simulink model "Main_v2"  (R2022b)
settings: Solver=ode23  StartTime=0.0  StopTime=sim_time-0.02
values from neighbouring files (symbols this model uses):
  bike_model = 1    [Main_sim.m]    (also in Startup_Script.m; Startup_Script_v2.m)
  bike_params = LoadBikeParameters(bike)    [Kalman_offline.m]    (also in Main_sim.m; Startup_Script.m; Startup_Script_v2.m; Startup_labview.m)
  C1 = [1 0 0 0 0 0 0 ... (first row only)    [Kalman_offline.m]    (also in Main_sim.m; Startup_Script.m; Startup_Script_v2.m; Startup_labview.m)
  counter = (Ts_GPS / Ts) - 1    (= 9)    [Kalman_offline.m]    (also in Main_sim.m; Startup_Script.m; Startup_Script_v2.m; Startup_labview.m)
  D_balancing_inner = 0    [Main_sim.m]    (also in Startup_Script.m; Startup_Script_v2.m; Startup_labview.m)
  D_balancing_outer = 0.0    (= 0)    [Main_sim.m]    (also in Startup_Script.m; Startup_Script_v2.m; Startup_labview.m)
  e1_max = abs(-k2*e2_max/k1)    [Main_sim.m]    (also in Startup_Script.m; Startup_Script_v2.m; Startup_labview.m)
  g = -9.81    [Kalman_offline.m]    (also in Main_sim.m = 9.81; Startup_Script.m = 9.81; Startup_Script_v2.m = 9.81; Startup_labview.m = 9.81)
  hor_dis = 10    [Main_sim.m]    (also in Startup_Script.m = 1; Startup_Script_v2.m = 1)
  I_balancing_inner = 0    [Main_sim.m]    (also in Startup_Script.m; Startup_Script_v2.m; Startup_labview.m)
  I_balancing_outer = 0.0    (= 0)    [Main_sim.m]    (also in Startup_Script.m; Startup_Script_v2.m; Startup_labview.m)
  initial_state_estimate = initial_state    [Main_sim.m]    (also in Startup_Script.m; Startup_Script_v2.m)
  k1 = K(1)    [Main_sim.m]    (also in Startup_Script.m; Startup_Script_v2.m; Startup_labview.m)
  k2 = K(2)    [Main_sim.m]    (also in Startup_Script.m; Startup_Script_v2.m; Startup_labview.m)
  Kalman_gain1 = Kalman_gain1'    [Kalman_offline.m]    (also in Main_sim.m; Startup_Script.m; Startup_Script_v2.m; Startup_labview.m)
  Kalman_gain2 = Kalman_gain2'    [Kalman_offline.m]    (also in Main_sim.m = Kalman_gain1(4:7,3:7); Startup_Script.m; Startup_Script_v2.m; Startup_labview.m = Kalman_gain1(4:7,3:7))
  linearized_sys = ss(A,B,C,D)    [Startup_Script_v2.m]
  P_balancing_inner = 3    [Main_sim.m]    (also in Startup_Script.m; Startup_Script_v2.m; Startup_labview.m = 1)
  P_balancing_outer = 1.3    [Main_sim.m]    (also in Startup_Script.m; Startup_Script_v2.m; Startup_labview.m = 1.75)
  Psiref = psiref'    [ReferenceGenerator.m]
  ref_dis = 0.01    [Main_sim.m]    (also in Startup_Script.m; Startup_Script_v2.m)
  ref_start_idx = 2    [Main_sim.m]    (also in Startup_Script.m; Startup_Script_v2.m)
  Ts = 0.01    [Kalman_offline.m]    (also in Main_sim.m; Startup_Script.m; Startup_Script_v2.m; Startup_labview.m)
  v = 3    [Main_sim.m]    (also in Startup_Script.m; Startup_Script_v2.m; Startup_labview.m = 2; Test_ss.m)
  Xref = xref'    [ReferenceGenerator.m]
  Yref = yref'    [ReferenceGenerator.m]
undefined symbols (not defined in the file or in its folder): initial_state, pert_deltadot_state, pert_deltadot_state_fun, pert_phidot_state, pert_phidot_state_fun
libraries: eeGeneralControl x3, slpidlib x2, simulink x2, cstblocks x1
(part 2 of 2)

== matlab function Main_v2/State estimator/Linearized Bicycle Model on Constant Velocity ==
  data: Est_States input; dot_delta_e input; y input; Kalman_gain1 input; Kalman_gain2 input; bike_params input; Ts input; Est_states output; v input; flag input
function Est_states  = fcn(Est_States, dot_delta_e, y, Kalman_gain1, Kalman_gain2, bike_params,Ts,v,flag)
% description 
% Inputs
%   Est_States := [X Y psi phi phi_dot delta_e v] are global at time t 
%   dot_delta_e := effective steering rate
%   y := measurement vector
%   Kalman_gain1 := Computed state_feedback gain including GPS meas
%   Kalman_gain2 := Computed state_feedback gain excluding GPS meas
%   bike_params := vector of bike parameters + gravity
%   Ts := Estimator sampling rate
%   v := constant velocity
%   flag := [0-1] increasing counter reseted at 1. When flag == 0 means
%           that GPS measurement is available
%
% Outputs
%   Est_states : = [X Y psi phi phi_dot delta_e v] global at time t+1

% Unpacked bike_params
    g = bike_params(1);
    h = bike_params(2);
    b = bike_params(3);
    a = bike_params(4);
    lambda = bike_params(5);
    c = bike_params(6);
    m = bike_params(7);
    h_imu = bike_params(8);

% Paper symbology
    lr = a; % distance from rear wheel center to center of mass
    lf = b-a; % distance from front wheel center to center of mass


% Transform the states to local frame 
    Est_States_l = zeros(7,1);
    
    Est_States_l(1) = Est_States(1) * cos(Est_States(3)) + Est_States(2) * sin(Est_States(3));
    Est_States_l(2) = -Est_States(1) * sin(Est_States(3)) + Est_States(2) * cos(Est_States(3));
    Est_States_l(3) = 0;        % direction of bike is aligned with X local frame
    Est_States_l(4) = Est_States(4);
    Est_States_l(5) = Est_States(5);
    Est_States_l(6) = Est_States(6);
    Est_States_l(7) = Est_States(7);

% Transform measurements to local frame
    y_l = zeros(size(y));

    y_l(1) = y(1) * cos(Est_States(3)) + y(2) * sin(Est_States(3));
    y_l(2) = -y(1) * sin(Est_States(3)) + y(2) * cos(Est_States(3)); 
    y_l(3) = y(3);
    y_l(4) = y(4);
    y_l(5) = y(5);
    y_l(6) = y(6);
    y_l(7) = y(7);


% % Continuous Time update in local frame TODO: x(t+1) = (I+A delta_T)h_hat(t)
%     states_dot = zeros(7,1);
%     
%     states_dot(1) = Est_States(7);
%     states_dot(2) = v * (Est_States_l(3) + (lr/(lr+lf))*Est_States(6) );
%     states_dot(3) = (v/(lr+lf)) * Est_States(6);
%     states_dot(4) = Est_States(5);
%     states_dot(5) = (g/h)*Est_States(4) + ((v^2*h-lr*g*c)/(h*(lr+lf)))*Est_States(6) + ((lr*v)/(h^2*(lr+lf)))*dot_delta_e;
%     states_dot(6) = dot_delta_e;
%     states_dot(7) = 0;
% 
% % Discrete time update in local 
%     Est_States_l = Est_States_l + states_dot * Ts; 

% % C identity is used to see if the code runs
%     sen = zeros(6,1);
%     sen(1)      = States_l(1);  
%     sen(2)      = States_l(2);
%     %sen(3)      = States_l(3);
%     sen(3)      = States_l(4);
%     sen(4)      = States_l(5);
%     sen(5)      = States_l(6);
%     sen(6)      = States_l(7);

% % Transform measurements into local frame to see if code runs
%     meas_l = zeros(6,1);
%     meas_l(1) = meas(1) * cos(States(3)) + meas(2) * sin(States(3));
%     meas_l(2) = -meas(1) * sin(States(3)) + meas(2) * cos(States(3));
%     meas_l(3) = 0;
%     meas_l(3) = meas(3)-States(3);  
%     meas_l(3) = meas(4);
%     meas_l(4) = meas(5);
%     meas_l(5) = meas(6);
%     meas_l(6) = meas(7);
%     meas_l(7) = meas(7);

% Time update in local frame (from t to t+1)
    % A matrix (linear bicycle model with constant velocity)
    A = [0 0 0 0 0 0 1;
         0 0 v 0 0 v*(lr/(lf+lr)) 0;
         0 0 0 0 0 (v/(lr+lf)) 0;
         0 0 0 0 1 0 0;
         0 0 0 (g/h) 0 ((v^2*h-lr*g*c)/(h^2*(lr+lf))) 0;
         0 0 0 0 0 0 0;
         0 0 0 0 0 0 0];
    
    % B matrix (linear bicycle model with constant velocity)
    B = [0 0 0 0 ((lr*v)/(h*(lr+lf))) 1 0]';
    
    % Discretization
    A_d = (eye(size(A))+Ts*A);
    B_d = Ts*B;

    % Time update
     Est_States_l = A_d*Est_States_l + B_d*dot_delta_e;

% Measurement update in local frame
    Est_states_l = zeros(7,1);

    % Sampling differentiation (Sensors rate 100Hz but GPS 10Hz)

    if flag == 0 % GPS sensors included
    
        % Select Kalman Gain
            K = Kalman_gain1;
    
        % C matrix for measurements
            X_GPS       = Est_States_l(1);  
            Y_GPS       = Est_States_l(2);
            a_y         = Est_States_l(6)*((-h_imu*(h*v^2-(g*a*c))*sin(lambda)/(b*h^2))+((v^2*sin(lambda))/(b))) + Est_States_l(4)*(g-((h_imu*g)/(h)))+ (-h_imu*a*v*sin(lambda)/(b*h))*dot_delta_e;
            omega_x     = Est_States_l(5);
            omega_z     = Est_States_l(6)*(v*sin(lambda))/(b);
            delta_enc   = Est_States_l(6);
            v_sens      = Est_States_l(7);
            y_pred = [X_GPS Y_GPS a_y omega_x omega_z delta_enc v_sens]';
    
        % Measurement update
            Est_states_l = Est_States_l + K * (y_l - y_pred);
            
    else % GPS sensors excluded
    
        % Select Kalman Gain
            K = Kalman_gain2;
    
        % C matrix for measurements
            a_y         = Est_States_l(6)*((-h_imu*(h*v^2-(g*a*c))*sin(lambda)/(b*h^2))+((v^2*sin(lambda))/(b))) + Est_States_l(4)*(g-((h_imu*g)/(h)))+ (-h_imu*a*v*sin(lambda)/(b*h))*dot_delta_e;
            omega_x     = Est_States_l(5);
            omega_z     = Est_States_l(6)*(v*sin(lambda))/(b);
            delta_enc   = Est_States_l(6);
            v_sens      = Est_States_l(7);
            y_pred = [a_y omega_x omega_z delta_enc v_sens]';
            
        % Measurement update
        Est_states_l(1) = Est_States_l(1);
        Est_states_l(2) = Est_States_l(2);
        Est_states_l(3) = Est_States_l(3);
        Est_states_l(4) = Est_States_l(4)+ K(1,:) * (y_l(3:7) - y_pred);
        Est_states_l(5) = Est_States_l(5) ;%+ K(2,:) * (y_l(3:7) - y_pred);
        Est_states_l(6) = Est_States_l(6)+ K(3,:) * (y_l(3:7) - y_pred);
        Est_states_l(7) = Est_States_l(7)+ K(4,:) * (y_l(3:7) - y_pred);

%         Est_states_l(4:7) = Est_States_l(4:7) + K * (y_l(3:7) - y_pred);
    end

    % states_l = Kalman_gain * (meas_l - sen);
    % states_l(1) = States_l(1) + Kalman_gain(1,1) * (meas_l(1) - x_m) + Kalman_gain(1,2) * (meas_l(2) - y_m) + Kalman_gain(1,3) * (meas_l(3) - psi_m) + Kalman_gain(1,4) * (meas_l(4) - phi_m) + Kalman_gain(1,5) * (meas_l(5) - dot_phi_m) + Kalman_gain(1,6) * (meas_l(6) - delta_m) + Kalman_gain(1,7) * (meas_l(7) - v_m);
    % states_l(2) = States_l(2) + Kalman_gain(2,1) * (meas_l(1) - x_m) + Kalman_gain(2,2) * (meas_l(2) - y_m) + Kalman_gain(2,3) * (meas_l(3) - psi_m) + Kalman_gain(2,4) * (meas_l(4) - phi_m) + Kalman_gain(2,5) * (meas_l(5) - dot_phi_m) + Kalman_gain(2,6) * (meas_l(6) - delta_m) + Kalman_gain(2,7) * (meas_l(7) - v_m);
    % states_l(3) = States_l(3) + Kalman_gain(3,1) * (meas_l(1) - x_m) + Kalman_gain(3,2) * (meas_l(2) - y_m) + Kalman_gain(3,3) * (meas_l(3) - psi_m) + Kalman_gain(3,4) * (meas_l(4) - phi_m) + Kalman_gain(3,5) * (meas_l(5) - dot_phi_m) + Kalman_gain(3,6) * (meas_l(6) - delta_m) + Kalman_gain(3,7) * (meas_l(7) - v_m);
    % states_l(4) = States_l(4) + Kalman_gain(4,1) * (meas_l(1) - x_m) + Kalman_gain(4,2) * (meas_l(2) - y_m) + Kalman_gain(4,3) * (meas_l(3) - psi_m) + Kalman_gain(4,4) * (meas_l(4) - phi_m) + Kalman_gain(4,5) * (meas_l(5) - dot_phi_m) + Kalman_gain(4,6) * (meas_l(6) - delta_m) + Kalman_gain(4,7) * (meas_l(7) - v_m);
    % states_l(5) = States_l(5) + Kalman_gain(5,1) * (meas_l(1) - x_m) + Kalman_gain(5,2) * (meas_l(2) - y_m) + Kalman_gain(5,3) * (meas_l(3) - psi_m) + Kalman_gain(5,4) * (meas_l(4) - phi_m) + Kalman_gain(5,5) * (meas_l(5) - dot_phi_m) + Kalman_gain(5,6) * (meas_l(6) - delta_m) + Kalman_gain(5,7) * (meas_l(7) - v_m);
    % states_l(6) = States_l(6) + Kalman_gain(6,1) * (meas_l(1) - x_m) + Kalman_gain(6,2) * (meas_l(2) - y_m) + Kalman_gain(6,3) * (meas_l(3) - psi_m) + Kalman_gain(6,4) * (meas_l(4) - phi_m) + Kalman_gain(6,5) * (meas_l(5) - dot_phi_m) + Kalman_gain(6,6) * (meas_l(6) - delta_m) + Kalman_gain(6,7) * (meas_l(7) - v_m);
    % states_l(7) = States_l(7) + Kalman_gain(7,1) * (meas_l(1) - x_m) + Kalman_gain(7,2) * (meas_l(2) - y_m) + Kalman_gain(7,3) * (meas_l(3) - psi_m) + Kalman_gain(7,4) * (meas_l(4) - phi_m) + Kalman_gain(7,5) * (meas_l(5) - dot_phi_m) + Kalman_gain(7,6) * (meas_l(6) - delta_m) + Kalman_gain(7,7) * (meas_l(7) - v_m);

% Transform to global the local states at time t+1 after measurement update
    Est_states = zeros(7,1);
    Est_states(3) = Est_States(3) + Est_states_l(3);    % direction update global
    
    % Change of Coordinates from local to global frame for  states 
    Est_states(1) = Est_states_l(1) * cos(Est_States(3)) - Est_states_l(2) * sin(Est_States(3));
    Est_states(2) = Est_states_l(1) * sin(Est_States(3)) + Est_states_l(2) * cos(Est_States(3));
    Est_states(4) = Est_states_l(4);
    Est_states(5) = Est_states_l(5);
    Est_states(6) = Est_states_l(6);
    Est_states(7) = Est_states_l(7);
    
    % Heading angle between pi and -pi
    Est_states(3) = wrapToPi(Est_states(3));

end

== matlab function Main_v2/Unstable bike model/Track bycicle pose/Derivative of positions ==
  data: Speed input; beta input; psi input; Xdot output; Ydot output
function [Xdot, Ydot]  = fcn(Speed, beta, psi)

Xdot = Speed * cos(psi + beta);
Ydot = Speed * sin(psi + beta);

== matlab function Main_v2/Unstable bike model/Nonlinear Model of the Physical Bicycle/MATLAB Function ==
  data: States input; xdot output; Steering_rate input; Speed input; disturbances input; bike_params input
function xdot = fcn(States, Steering_rate, Speed, disturbances, bike_params)
% Unpacked bike_params
    g = bike_params(1);
    h = bike_params(2);
    b = bike_params(3);
    a = bike_params(4);
    lambda = bike_params(5);
    c = bike_params(6);
    m = bike_params(7);
    h_imu = bike_params(8);

% Paper symbology
    lr = a; % distance from rear wheel center to center of mass
    lf = b-a; % distance from front wheel center to center of mass

d_phidot = disturbances(1);
d_deltadot = disturbances(2);

phi = States(1);
delta = States(2);
phi_d = States(3);

% xdot = [phidot deltadot phiddot]
xdot1 = phi_d + d_phidot;
xdot2 = Steering_rate + d_deltadot;
xdot3 = (g/h)*phi + ((lr*Speed*sin(lambda))/((lr+lf)*h))*Steering_rate + ((h*Speed^2-g*lr*c)/((lr+lf)*h^2))*sin(lambda)*delta;

xdot = [xdot1 xdot2 xdot3]';

== matlab function Main_v2/Trajectory controller (error based)/Trajectory controller (Error based) ==
  data: k1 input; k2 input; e1 input; e2 input; steer_angle output; e1_max input
function steer_angle = fcn(k1,k2,e1,e2,e1_max)

% Errors are based on distance error and heading error (true position and heading with respect to closest reference position and heading)
delta=-k1*sign(e1)*min(abs(e1),e1_max)-k2*e2;

steer_angle = delta;

== matlab function Main_v2/Unstable bike model/Track bycicle pose/MATLAB Function ==
  data: Speed input; beta output; Steering input; bike_params input; psi_dot output
function [beta, psi_dot] = fcn(Speed, Steering, bike_params)
a       = bike_params(1);
b       = bike_params(2);
lambda  = bike_params(3);

eff_steering = sin(lambda) * Steering;

beta = atan(a /b * tan(eff_steering) );
psi_dot = (Speed / a) * sin(beta);

== matlab function Main_v2/Sensors/Define true sensor positions on the bike ==
  data: bike_params input; pose input; pose_corrected output
function pose_corrected  = fcn(bike_params, pose)
pose_corrected = pose;

gpsX = bike_params(1); % measured offset of GPS parallel to bike
gpsY = bike_params(2); % measured offset of GPS perpendicular to bike
gpsH = bike_params(3); % measured offset of GPS from ground to GPS

% define pose_l
pose_l = pose;

% Transform to local frame
    pose_l(1) =  pose(1) * cos(pose(3)) + pose(2) * sin(pose(3));
    pose_l(2) = -pose(1) * sin(pose(3)) + pose(2) * cos(pose(3)); 

% define actual positions of GPS 
% pose1 = difference in x in local frame
% pose2 = difference in y in local frame
    pose_l(1) = pose_l(1) + gpsX;
    pose_l(2) = pose_l(2) + gpsY + gpsH*sin(pose(4));

% define actual positions of IMU 


% Transform back to global frame
    pose(1) = pose_l(1) * cos(pose(3)) - pose_l(2) * sin(pose(3));
    pose(2) = pose_l(1) * sin(pose(3)) + pose_l(2) * cos(pose(3));

pose_corrected(1) = pose(1);
pose_corrected(2) = pose(2);

== matlab function Main_v2/Unstable bike model/Nonlinear Model of the Physical Bicycle/Nonlinear Bicycle Model without front wheel inertia ==
  data: States input; Steering_rate input; Speed input; disturbances input; xdot output; Parameters parameter
function xdot = fcn(States, Steering_rate, Speed, disturbances, Parameters)

g = 9.81;

d_phidot = disturbances(1);
d_deltadot = disturbances(2);

phi = States(1);
delta = States(2);
phi_d = States(3);

% xdot = [phidot deltadot phiddot]
xdot1 = phi_d + d_phidot;
xdot2 = Steering_rate + d_deltadot;
xdot3 = (g/Parameters.h)*sin(phi) + ((Parameters.a*Speed)/(Parameters.b*Parameters.h))/(cos(sin(Parameters.lambda)*delta)^2)*sin(Parameters.lambda)*Steering_rate ...
                                  + ((Parameters.h*Speed^2-g*Parameters.a*Parameters.c)/(Parameters.b*Parameters.h^2))*sin(Parameters.lambda)*tan(delta);

xdot = [xdot1 xdot2 xdot3]';

== matlab function Main_v2/Closest point algorithm & Error calculation/Closest point algorithm & Error calculation ==
  settings: updateMethod=DISCRETE  sampleTime=Ts
  data: e1 output; e2 output; dpsiref output; closestpoint_idx output; closestpoint_heading_idx output; Xref_loc input; Yref_loc input; psiref_loc input; X_est input; Y_est input; psi_est input; ref_X output; ref_Y output; ref_psi output; v input
function [e1,e2,dpsiref,closestpoint_idx,closestpoint_heading_idx,ref_X,ref_Y,ref_psi]= fcn(Xref_loc,Yref_loc,psiref_loc,X_est,Y_est,psi_est,v)
%% calculations on a local part of the trajectory

% Each referencepoint has a location (X,Y) and a heading
% The heading is defined in the startup.m file as 'the heading where its coming from' 
% Second point in local reference is current selected closest point
closestpoint_idx=2;

% Search for closest point
% Finding the closest point going forward. Stop searching once next
% distance increases

while (Xref_loc(closestpoint_idx,1)-X_est)^2 + (Yref_loc(closestpoint_idx,1)-Y_est)^2 >= (Xref_loc(closestpoint_idx+1,1)-X_est)^2+(Yref_loc(closestpoint_idx+1,1)-Y_est)^2  && closestpoint_idx <= length(Xref_loc)-2
closestpoint_idx = closestpoint_idx+1;
end

% Select same closest point (for heading error and position error)
closestpoint_heading_idx = closestpoint_idx;


% Calculate X and Y distance from current location to selected closest
% point
dx = X_est - Xref_loc(closestpoint_idx,1);
dy = Y_est - Yref_loc(closestpoint_idx,1);

% Calculate difference in current heading and heading in reference point 
% And limit D_psiref  between -2pi and 2pi
D_psiref=psiref_loc(closestpoint_idx+1,1)-psiref_loc(closestpoint_idx,1);
if D_psiref>=pi
    D_psiref=mod(D_psiref,-2*pi);
end
if D_psiref<=-pi
    D_psiref=mod(D_psiref,2*pi);
end

%IMPROVEMENT: implement an interpolation algoritm
% Calculate distence between point before closest point and current location
dist_true_previous = sqrt((Xref_loc(closestpoint_idx-1,1)-X_est)^2+(Yref_loc(closestpoint_idx-1,1)-Y_est)^2);
% Angle of line between previous closest point and current location
alpha_star = atan((Yref_loc(closestpoint_idx-1,1)-Y_est)/(Xref_loc(closestpoint_idx-1,1)-X_est));
% heading previous closest point - alpha star
alpha_projected_dist = alpha_star-psiref_loc(closestpoint_idx,1);
% the distance from the previous closest point to the projection of the bike on the trajectory
Projected_dist = dist_true_previous*cos(alpha_projected_dist);

compared_dist = sqrt((Xref_loc(closestpoint_idx,1)-Xref_loc(closestpoint_idx-1,1))^2+(Yref_loc(closestpoint_idx,1)-Yref_loc(closestpoint_idx-1,1))^2);

% OLD: Calculate lateral distance from current position to trajectory with current heading
% e1_prev = dy*cos(psiref_loc(closestpoint_idx,1)) - dx*sin(psiref_loc(closestpoint_idx,1));
% Projected_dist =  dist_true_previous^2-e1_prev^2;

% If bike passes closest point, the heading of the next point will be taken
if Projected_dist >= compared_dist
closestpoint_heading_idx = closestpoint_idx+1;
end

%calculate e1 and e2        
e1= dy*cos(psiref_loc(closestpoint_heading_idx,1)) - dx*sin(psiref_loc(closestpoint_heading_idx,1)); % this make e1 include "direction" automatically
e2= psi_est-psiref_loc(closestpoint_heading_idx,1); %calculate e2

% closest point on the local trajectory
ref_X=Xref_loc(closestpoint_idx,1);
ref_Y=Yref_loc(closestpoint_idx,1);
ref_psi=psiref_loc(closestpoint_idx,1);

 % keep heading error should be between -pi 2 pi
e2 = wrapToPi(e2);
%e2=mod(e2+pi,2*pi)-pi;     

%calculate the time between psiref(idx,1) and psiref(idx+1,1)
dX=Xref_loc(closestpoint_idx+1,1)-ref_X;
dY=Yref_loc(closestpoint_idx+1,1)-ref_Y;
dis=sqrt(dX^2+dY^2);
Ts_psi=dis/v;

% Sample dpsiref
dpsiref=(D_psiref)/Ts_psi;

% Reset closest point index as feedback for local frame selection
closestpoint_idx = closestpoint_idx-1;

end

== matlab function Main_v2/convert steer angle into ref roll/Convert steer angle to roll ==
  data: steer_angle_ref input; roll_ref output; bike_params input; v input
function roll_ref = fcn(steer_angle_ref, bike_params, v)

lambda = bike_params(1);
b      = bike_params(2);
g      = bike_params(3);

eff_steer_angle = -1*atan((tan(steer_angle_ref*sin(lambda))*(v^2/b))/g);

roll_ref = eff_steer_angle;
